simulink model "multi_model_attitude_controller1_1"  (R2016b)
settings: Solver=ode15s  StartTime=0.0  StopTime=inf  FixedStep=0.001  MaxStep=0.004  RelTol=1e-3
InitFcn:
  | kR_old=0;
  | kOm_old=0;
undefined symbols (not defined in the file or in its folder): deg, rad, s
libraries: simulink x32, aerolibconvert2 x6, aerolibobsolete x2, aerolibtransform2 x2, aerolibatmos2 x2, aerolibnav x2, aerolibanimutils x2
(part 1 of 3)
settings Model: Creator=ADAM  LastModifiedBy=luminghua
settings SolverCC: ExtrapolationOrder=1
settings DataIOCC: MaxDataPoints=1  SaveFormat=Structure  SignalLoggingSaveFormat=ModelDataLogs  SaveOutput=off  SignalLogging=off  DSMLogging=off  SaveTime=off  OutputSaveName=model_out  SignalLoggingName=model_out
settings OptimizationCC: ExpressionDepthLimit=2147483647  LifeSpan=inf  SimCompilerOptimization=on
settings DebuggingCC: UnderspecifiedInitializationDetection=Classic  MergeDetectMultiDrivingBlocksExec=none  SolverPrmCheckMsg=warning  InheritedTsInSrcMsg=none  MultiTaskDSMMsg=warning  MultiTaskCondExecSysMsg=none  FcnCallInpInsideContextMsg=warning  UnconnectedInputMsg=none  UnconnectedOutputMsg=none  UnconnectedLineMsg=none  AllowSymbolicDim=off  StateNameClashWarn=warning  SFUnexpectedBacktrackingDiag=warning  SFNoUnconditionalDefaultTransitionDiag=warning  SFExecutionAtInitializationDiag=none
settings HardwareCC: ProdBitPerPointer=32  ProdBitPerSizeT=32  ProdBitPerPtrDiffT=32  ProdLargestAtomicFloat=None  ProdWordSize=32  ProdHWDeviceType=Generic->32-bit x86 compatible
settings ModelReferenceCC: PropagateSignalLabelsOutOfModel=off
settings CodeAppCC: MaxIdLength=95
settings GRTTargetCC: TargetLangStandard=C89/C90 (ANSI)  GeneratePreprocessorConditionals=Disable all
settings ConfigComp: CovMetricSettings=dw  CovHtmlReporting=on  CovSaveCumulativeToWorkspaceVar=on  CovSaveSingleToWorkspaceVar=on  CovExternalEMLEnable=off

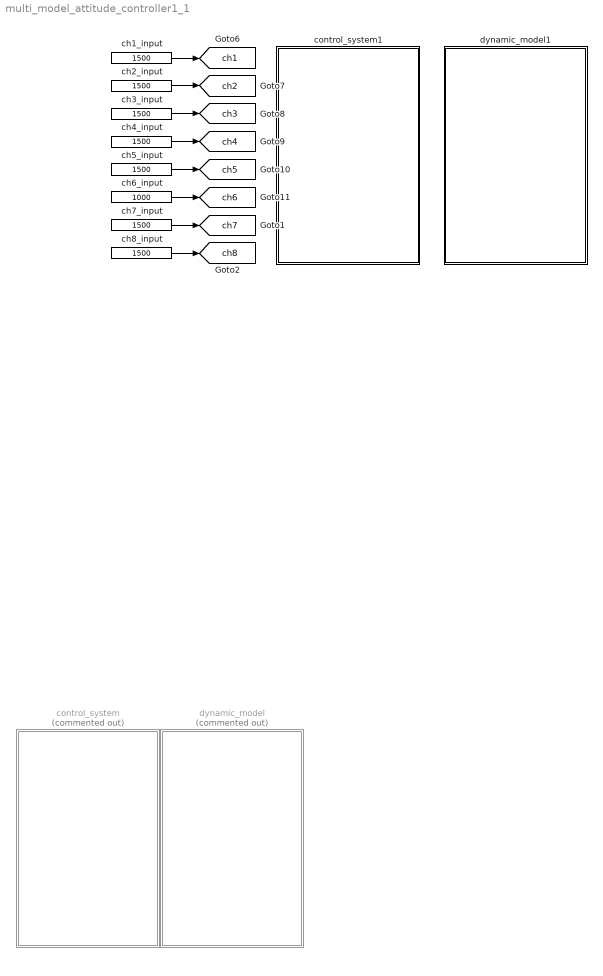
== system multi_model_attitude_controller1_1 ==
  ch1_input : Constant  Value=1500  SampleTime=0.004
  ch2_input : Constant  Value=1500  SampleTime=0.004
  ch3_input : Constant  Value=1500  SampleTime=0.004
  ch4_input : Constant  Value=1500  SampleTime=0.004
  ch5_input : Constant  Value=1500  SampleTime=0.004
  ch6_input : Constant  Value=1000  SampleTime=0.004
  ch7_input : Constant  Value=1500  SampleTime=0.004
  ch8_input : Constant  Value=1500  SampleTime=0.004
  control_system : Subsystem  Commented=on
      mask Display: fprintf('Embedded Software')
  control_system1 : Subsystem
      mask Display: fprintf('Embedded Software')
  dynamic_model : Subsystem  Commented=on
      mask Display: fprintf('Dynamic Model');
  dynamic_model1 : Subsystem
      mask Display: fprintf('Dynamic Model');
  tag scope: ch1=global, ch2=global, ch3=global, ch4=global, ch5=global, ch6=global, ch7=global, ch8=global
  wires:
  ch3_input/1 -> [ch3]
  ch2_input/1 -> [ch2]
  ch1_input/1 -> [ch1]
  ch4_input/1 -> [ch4]
  ch5_input/1 -> [ch5]
  ch6_input/1 -> [ch6]
  ch7_input/1 -> [ch7]
  ch8_input/1 -> [ch8]

== system multi_model_attitude_controller1_1/control_system ==
  Constant4 : Constant  Commented=on  Value=0.07  SampleTime=0.004
  Constant6 : Constant  Commented=on  Value=0  SampleTime=0.004
  Constant7 : Constant  Commented=on  Value=0  SampleTime=0.004
  Fcn2 : Fcn  Expr=(u - 1500) / 500
  Fcn5 : Fcn  Expr=(u - 1500) / 500
  Fcn6 : Fcn  Expr=(u - 1000) / 1000
  Fcn7 : Fcn  Expr=(u - 1500) / 500
  Mux : Mux  Inputs=3
  Saturation10 : Saturate  UpperLimit=1  LowerLimit=0
  Saturation7 : Saturate  UpperLimit=1  LowerLimit=-1
  Saturation8 : Saturate  UpperLimit=1  LowerLimit=-1
  Saturation9 : Saturate  UpperLimit=1  LowerLimit=-1
  Subsystem : Subsystem
      mask Display: disp('Test')
  Subsystem1 : Subsystem  Commented=on
      mask Display: disp('Attitude_controller distur');
  Subsystem2 : Subsystem  Commented=on
      mask Display: disp( 'Attitude_controller  PID')
  Subsystem3 : Subsystem
      mask Display: disp('Attitude_controller distur');
  tag scope: Moment=global
  wires:
  [ch1] -> Fcn2/1
  [ch2] -> Fcn5/1
  [ch4] -> Fcn7/1
  Fcn7/1 -> Saturation7/1
  Fcn5/1 -> Saturation8/1
  Fcn2/1 -> Saturation9/1
  [ch3] -> Fcn6/1
  Fcn6/1 -> Saturation10/1
  Subsystem1/1(M_roll) -> ?  "M_roll"
  Subsystem1/2(M_pitch) -> ?  "M_pitch"
  Subsystem1/3(M_yaw) -> ?  "M_yaw"
  Subsystem2/1(Out1) -> ?  "M_roll"
  Subsystem2/2(Out2) -> ?  "M_pitch"
  Subsystem2/3(Out3) -> ?  "M-yaw"
  Constant7/1 -> ?
  Constant6/1 -> ?
  Constant4/1 -> ?
  Subsystem3/1(M_roll) -> Mux/1
  Subsystem3/2(M_pitch) -> Mux/2
  Subsystem3/3(M_yaw) -> Mux/3
  Mux/1 -> [Moment]

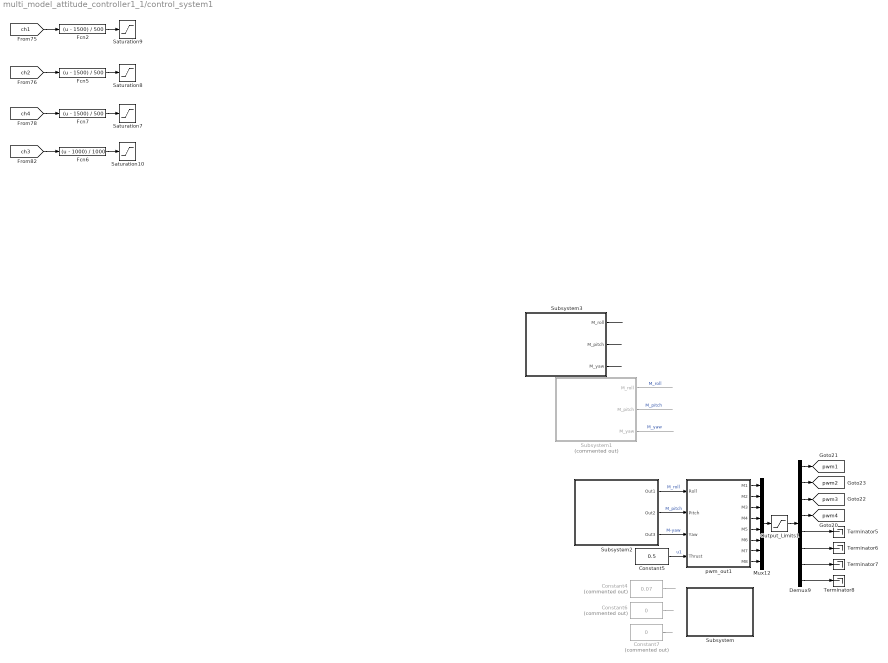
== system multi_model_attitude_controller1_1/control_system1 ==
  Constant4 : Constant  Commented=on  Value=0.07  SampleTime=0.004
  Constant5 : Constant  Value=0.5  SampleTime=0.004
  Constant6 : Constant  Commented=on  Value=0  SampleTime=0.004
  Constant7 : Constant  Commented=on  Value=0  SampleTime=0.004
  Demux9 : Demux  Outputs=8
  Fcn2 : Fcn  Expr=(u - 1500) / 500
  Fcn5 : Fcn  Expr=(u - 1500) / 500
  Fcn6 : Fcn  Expr=(u - 1000) / 1000
  Fcn7 : Fcn  Expr=(u - 1500) / 500
  Mux12 : Mux  Inputs=8
  Output_Limits1 : Saturate  UpperLimit=2000  LowerLimit=1000
  Saturation10 : Saturate  UpperLimit=1  LowerLimit=0
  Saturation7 : Saturate  UpperLimit=1  LowerLimit=-1
  Saturation8 : Saturate  UpperLimit=1  LowerLimit=-1
  Saturation9 : Saturate  UpperLimit=1  LowerLimit=-1
  Subsystem : Subsystem
      mask Display: disp('Test')
  Subsystem1 : Subsystem  Commented=on
      mask Display: disp('Attitude_controller distur');
  Subsystem2 : Subsystem
      mask Display: disp( 'Attitude_controller  PID')
  Subsystem3 : Subsystem
      mask Display: disp('Attitude_controller distur');
  Terminator{5..8} (4 alike) : Terminator
  pwm_out1 : MATLAB Function  TreatAsAtomicUnit=on  SystemSampleTime=0.004
  tag scope: pwm1=global, pwm2=global, pwm3=global, pwm4=global
  wires:
  pwm_out1/8(M8) -> Mux12/8
  pwm_out1/7(M7) -> Mux12/7
  pwm_out1/6(M6) -> Mux12/6
  pwm_out1/5(M5) -> Mux12/5
  pwm_out1/4(M4) -> Mux12/4
  pwm_out1/3(M3) -> Mux12/3
  pwm_out1/2(M2) -> Mux12/2
  pwm_out1/1(M1) -> Mux12/1
  Mux12/1 -> Output_Limits1/1
  [ch1] -> Fcn2/1
  [ch2] -> Fcn5/1
  [ch4] -> Fcn7/1
  Fcn7/1 -> Saturation7/1
  Fcn5/1 -> Saturation8/1
  Fcn2/1 -> Saturation9/1
  Demux9/5 -> Terminator5/1
  Demux9/6 -> Terminator6/1
  Demux9/7 -> Terminator7/1
  Demux9/8 -> Terminator8/1
  Demux9/1 -> [pwm1]
  Demux9/2 -> [pwm2]
  Demux9/3 -> [pwm3]
  Demux9/4 -> [pwm4]
  [ch3] -> Fcn6/1
  Fcn6/1 -> Saturation10/1
  Output_Limits1/1 -> Demux9/1
  Constant5/1 -> pwm_out1/4(Thrust)  "u1"
  Subsystem1/1(M_roll) -> ?  "M_roll"
  Subsystem1/2(M_pitch) -> ?  "M_pitch"
  Subsystem1/3(M_yaw) -> ?  "M_yaw"
  Subsystem2/1(Out1) -> pwm_out1/1(Roll)  "M_roll"
  Subsystem2/2(Out2) -> pwm_out1/2(Pitch)  "M_pitch"
  Subsystem2/3(Out3) -> pwm_out1/3(Yaw)  "M-yaw"
  Constant7/1 -> ?
  Constant6/1 -> ?
  Constant4/1 -> ?
  Subsystem3/1(M_roll) -> ?
  Subsystem3/2(M_pitch) -> ?
  Subsystem3/3(M_yaw) -> ?

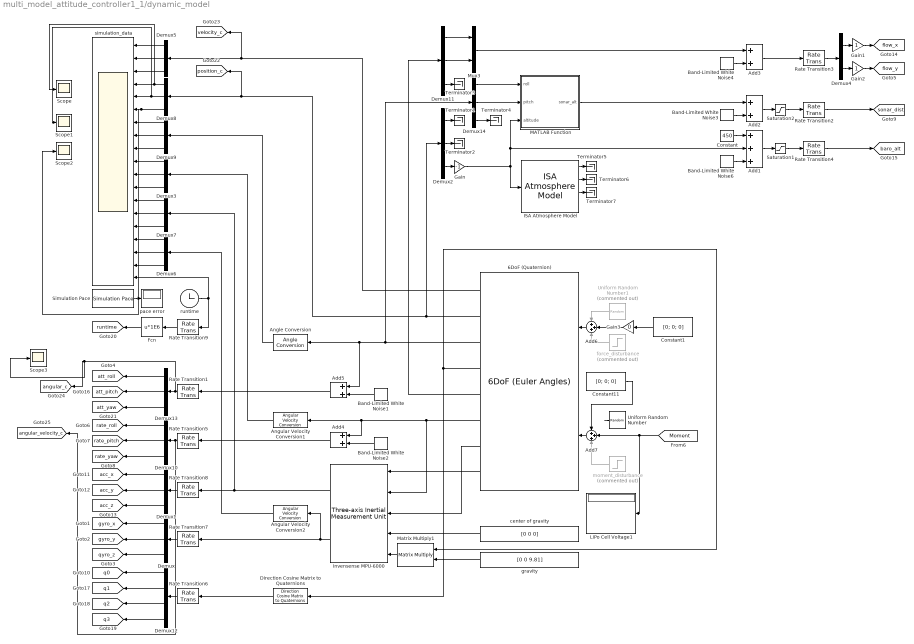
== system multi_model_attitude_controller1_1/dynamic_model ==
  6DoF (Quaternion) : aerolibobsolete/6DoF (Euler Angles)  units=Metric (MKS)  mtype=Fixed  rep=Quaternion  xme_0=[0 0 -1]  Vm_0=[0 0 0]  eul_0=[0 0 0]  pm_0=[0 0 0]  mass_0=0.26  mass_e=0  mass_f=0  inertia=[0.00080, 0, 0; 0, 0.00065, 0; 0, 0, 0.0014]  inertia_e=eye(3)  inertia_f=eye(3)  k_quat=1.0
  Add1 : Sum  Inputs=+++
  Add{2..5} (4 alike) : Sum
  Add6 : Sum  Inputs=+++
  Add7 : Sum  Inputs=+++
  Angle Conversion : aerolibconvert2/Angle Conversion  IU=rad  OU=deg
  Angular Velocity Conversion1 : aerolibconvert2/Angular Velocity Conversion  IU=rad/s  OU=deg/s
  Angular Velocity Conversion2 : aerolibconvert2/Angular Velocity Conversion  IU=rad/s  OU=deg/s
  Band-Limited White Noise1 : simulink/Sources/Band-Limited White Noise  Cov=0.00000000015  Ts=0.004  seed=[243584]
  Band-Limited White Noise2 : simulink/Sources/Band-Limited White Noise  Cov=0.000000002  Ts=0.004  seed=[243584]
  Band-Limited White Noise3 : simulink/Sources/Band-Limited White Noise  Cov=0.000005  Ts=0.1  seed=[31841]
  Band-Limited White Noise4 : simulink/Sources/Band-Limited White Noise  Cov=0.000000003  Ts=0.0067  seed=[25481]
  Band-Limited White Noise6 : simulink/Sources/Band-Limited White Noise  Cov=0.0005  Ts=0.008  seed=[79648]
  Constant : Constant  Value=450
  Constant1 : Constant  Value=[0; 0; 0]  SampleTime=5
  Constant11 : Constant  Value=[0; 0; 0]  SampleTime=5
  Demux{,1..3,5..11,13..14} (13 alike) : Demux  Outputs=3
  Demux12 : Demux
  Demux4 : Demux  Outputs=2
  Direction Cosine Matrix to Quaternions : aerolibtransform2/Direction Cosine Matrix  to Quaternions
  Fcn : Fcn  Expr=u*1E6
      mask Display: fprintf('uS');
  Gain : Gain  Gain=-1
  Gain1 : Gain
  Gain2 : Gain
  Gain3 : Gain  Gain=0
  ISA Atmosphere Model : aerolibatmos2/ISA Atmosphere Model  custom=on  g=9.80665  gamma=1.4  R=287.0531  L=0.0065  h_trop=11000  h_strat=20000  rho0=1.225  P0=101325  T0=288.15  h0=0
  Invensense MPU-6000 : aerolibnav/Three-axis Inertial Measurement Unit  units=Metric (MKS)  imu=[0 0 0]  i_Ts=0.004  dtype_a=off  w_a=190  z_a=0.707  a_sf_cc=[0.98 0 0; 0 0.98 0; 0 0 0.98]  a_bias=[0 0 0]  a_sat="[-19.62  -19.62  -19.62 19.62 19.62 19.62]"  dtype_g=off  w_g=190  z_g=0.707  g_sf_cc=[.98 0 0; 0 .98 0; 0 0 .98]  g_bias=[0 0 0]  g_sens=[0 0 0]  g_sat="[-4.36  -4.36  -4.36 4.36 4.36 4.36]"  i_rand=on  i_seeds=[348631 366719 978432 189621 128794 214632]  i_pow=[0.0000005 0.0000005 0.0000005 0.000000002 0.000000002 0.000000002]
  LiPo Cell Voltage1 : Display
  MATLAB Function : MATLAB Function  TreatAsAtomicUnit=on
  Matrix Multiply1 : Product  Multiplication=Matrix(*)
  Mux3 : Mux  Inputs=2
  Rate Transition{1,5..9} (6 alike) : RateTransition  OutPortSampleTime=0.004
  Rate Transition2 : RateTransition  OutPortSampleTime=0.1
  Rate Transition3 : RateTransition  OutPortSampleTime=0.0067
  Rate Transition4 : RateTransition  OutPortSampleTime=0.008
  Saturation1 : Saturate  UpperLimit=inf  LowerLimit=0
  Saturation2 : Saturate  UpperLimit=5  LowerLimit=0.3
  Scope{,1..3} (4 alike) : Scope
  Simulation Pace : aerolibanimutils/Simulation Pace  SimulationPace=1  SleepMode=MATLAB Thread  OutputPaceError=on  SampleTime=0.004
      settings: AttributesFormatString=%<SimulationPace> sec/sec
  Terminator{1..7} (7 alike) : Terminator
  Uniform Random Number : UniformRandomNumber  Minimum=[-0.0005 -0.0005 -0.0001]  Maximum=[0.5 0.0005 0.0001]  SampleTime=5
  Uniform Random Number1 : UniformRandomNumber  Commented=on  Minimum=[-0.01 -0.01 -0.1]  Maximum=[0.01 0.01 0.1]  SampleTime=5
  center of gravity : Constant  Value=[0 0 0]
  force_disturbance : Step  Commented=on  Time=5  Before=[0 0 0]  After=[0 0 0]
  gravity : Constant  Value=[0 0 9.81]
  moment_disturbance : Step  Commented=on  Time=5  Before=[0 0 0]  After=[0 0 0]
  pace error : Display
  runtime : Clock
  simulation_data : Scope  NumInputPorts=19
  tag scope: acc_x=global, acc_y=global, acc_z=global, angular_c=global, angular_velocity_c=global, att_pitch=global, att_roll=global, att_yaw=global, baro_alt=global, flow_x=global, flow_y=global, gyro_x=global, gyro_y=global, position_c=global, q0=global, q1=global, q2=global, q3=global, qyro_z=global, rate_pitch=global, rate_roll=global, rate_yaw=global, runtime=global, sonar_dist=global, velocity_c=global
  wires:
  6DoF (Quaternion)/7 -> Invensense MPU-6000/3
  Demux1/1 -> [acc_x]
  6DoF (Quaternion)/3 -> Demux14/1, Angle Conversion/1, Add5/1
  6DoF (Quaternion)/8 -> Invensense MPU-6000/1
  6DoF (Quaternion)/5 -> Demux11/1
  Demux9/1 -> simulation_data/7
  Demux9/2 -> simulation_data/8
  Demux3/1 -> simulation_data/10
  Demux3/2 -> simulation_data/11
  Demux3/3 -> simulation_data/12
  Demux7/1 -> simulation_data/13
  Demux7/2 -> simulation_data/14
  Demux7/3 -> simulation_data/15
  Demux/1 -> [gyro_x]
  Demux/2 -> [gyro_y]
  Demux/3 -> [qyro_z]
  Demux1/2 -> [acc_y]
  Demux5/1 -> simulation_data/1
  Demux5/2 -> simulation_data/2
  Demux5/3 -> simulation_data/3
  Demux8/1 -> Scope/1, simulation_data/4
  Demux8/2 -> Scope1/1, simulation_data/5
  Demux8/3 -> Scope2/1, simulation_data/6
  6DoF (Quaternion)/6 -> Invensense MPU-6000/2, Add4/1, Angular Velocity Conversion1/1
  Demux9/3 -> simulation_data/9
  Demux6/1 -> simulation_data/16
  Demux6/2 -> simulation_data/17
  Demux6/3 -> simulation_data/18
  Angular Velocity Conversion2/1 -> Demux6/1
  Demux1/3 -> [acc_z]
  Demux10/1 -> [rate_roll]
  Demux10/2 -> [rate_pitch]
  Demux10/3 -> [rate_yaw]
  Band-Limited White Noise2/1 -> Add4/2
  Add4/1 -> Rate Transition5/1
  Rate Transition5/1 -> [angular_velocity_c], Demux10/1
  6DoF (Quaternion)/4 -> Matrix Multiply1/1, Direction Cosine Matrix to Quaternions/1
  Simulation Pace/1 -> pace error/1
  6DoF (Quaternion)/1 -> Demux5/1, [velocity_c]
  6DoF (Quaternion)/2 -> Demux2/1, Demux8/1, [position_c]
  Angle Conversion/1 -> Demux9/1
  Angular Velocity Conversion1/1 -> Demux3/1
  Invensense MPU-6000/1 -> Rate Transition8/1, Demux7/1
  Invensense MPU-6000/2 -> Rate Transition7/1, Angular Velocity Conversion2/1
  runtime/1 -> simulation_data/19, Rate Transition9/1
  Rate Transition7/1 -> Demux/1
  Rate Transition8/1 -> Demux1/1
  Direction Cosine Matrix to Quaternions/1 -> Rate Transition6/1
  Rate Transition6/1 -> Demux12/1
  Demux12/4 -> [q3]
  Demux12/3 -> [q2]
  Demux12/2 -> [q1]
  Demux12/1 -> [q0]
  Fcn/1 -> [runtime]
  Rate Transition9/1 -> Fcn/1
  Demux13/1 -> [att_roll]
  Demux13/2 -> [att_pitch]
  Demux13/3 -> [att_yaw]
  Rate Transition1/1 -> Scope3/1, [angular_c], Demux13/1
  Band-Limited White Noise1/1 -> Add5/2
  Add5/1 -> Rate Transition1/1
  Add6/1 -> 6DoF (Quaternion)/1
  Add7/1 -> 6DoF (Quaternion)/2
  center of gravity/1 -> Invensense MPU-6000/4
  gravity/1 -> Matrix Multiply1/2
  Matrix Multiply1/1 -> Invensense MPU-6000/5
  moment_disturbance/1 -> Add7/3
  force_disturbance/1 -> Add6/3
  Constant1/1 -> Gain3/1
  Uniform Random Number1/1 -> Add6/1
  Uniform Random Number/1 -> ?
  Rate Transition3/1 -> Demux4/1
  Add3/1 -> Rate Transition3/1
  Demux2/3 -> Gain/1
  Gain/1 -> ISA Atmosphere Model/1, MATLAB Function/3(altitude), Add1/2
  Demux2/2 -> Terminator2/1
  Demux2/1 -> Terminator1/1
  Demux11/1 -> Mux3/1
  Demux11/2 -> Mux3/2
  Demux11/3 -> Terminator3/1
  Rate Transition2/1 -> [sonar_dist]
  Rate Transition4/1 -> [baro_alt]
  Saturation1/1 -> Rate Transition4/1
  Saturation2/1 -> Rate Transition2/1
  Add1/1 -> Saturation1/1
  MATLAB Function/1(sonar_alt) -> Add2/1
  Band-Limited White Noise3/1 -> Add2/2
  Add2/1 -> Saturation2/1
  Band-Limited White Noise4/1 -> Add3/2
  Band-Limited White Noise6/1 -> Add1/3
  Constant/1 -> Add1/1
  Mux3/1 -> Add3/1
  Demux4/2 -> Gain2/1
  Demux4/1 -> Gain1/1
  Gain1/1 -> [flow_x]
  Gain2/1 -> [flow_y]
  Demux14/2 -> MATLAB Function/2(pitch)
  Demux14/1 -> MATLAB Function/1(roll)
  Demux14/3 -> Terminator4/1
  ISA Atmosphere Model/3 -> Terminator7/1
  ISA Atmosphere Model/2 -> Terminator6/1
  ISA Atmosphere Model/1 -> Terminator5/1
  Constant11/1 -> Add7/1
  [Moment] -> Add7/2, LiPo Cell Voltage1/1
  Gain3/1 -> Add6/2

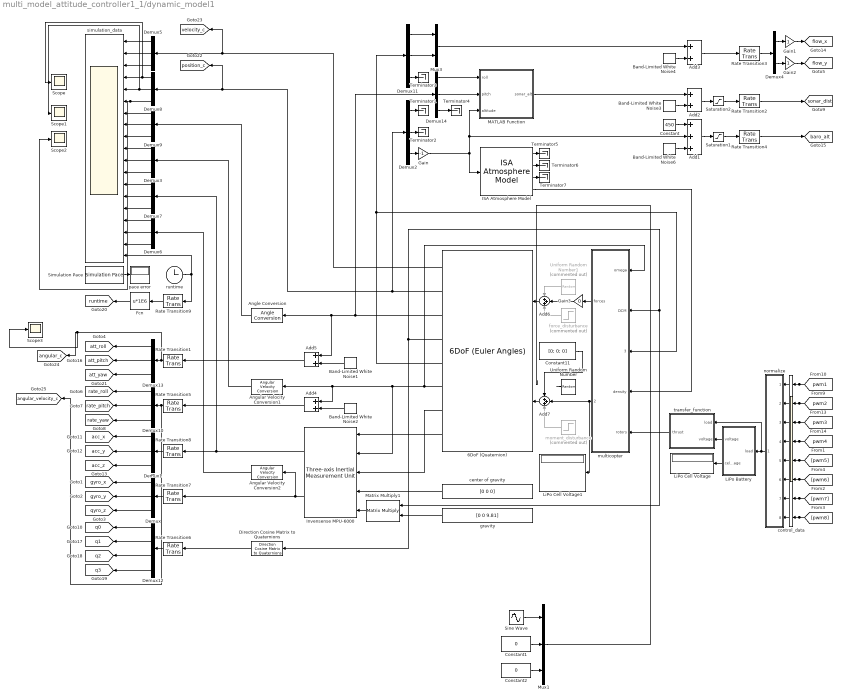
== system multi_model_attitude_controller1_1/dynamic_model1 ==
  6DoF (Quaternion) : aerolibobsolete/6DoF (Euler Angles)  units=Metric (MKS)  mtype=Fixed  rep=Quaternion  xme_0=[0 0 -1]  Vm_0=[0 0 0]  eul_0=[0 0 0]  pm_0=[0 0 0]  mass_0=0.26  mass_e=0  mass_f=0  inertia=[0.00080, 0, 0; 0, 0.00065, 0; 0, 0, 0.0014]  inertia_e=eye(3)  inertia_f=eye(3)  k_quat=1.0
  Add1 : Sum  Inputs=+++
  Add{2..5} (4 alike) : Sum
  Add6 : Sum  Inputs=+++
  Add7 : Sum  Inputs=+++
  Angle Conversion : aerolibconvert2/Angle Conversion  IU=rad  OU=deg
  Angular Velocity Conversion1 : aerolibconvert2/Angular Velocity Conversion  IU=rad/s  OU=deg/s
  Angular Velocity Conversion2 : aerolibconvert2/Angular Velocity Conversion  IU=rad/s  OU=deg/s
  Band-Limited White Noise1 : simulink/Sources/Band-Limited White Noise  Cov=0.00000000015  Ts=0.004  seed=[243584]
  Band-Limited White Noise2 : simulink/Sources/Band-Limited White Noise  Cov=0.000000002  Ts=0.004  seed=[243584]
  Band-Limited White Noise3 : simulink/Sources/Band-Limited White Noise  Cov=0.000005  Ts=0.1  seed=[31841]
  Band-Limited White Noise4 : simulink/Sources/Band-Limited White Noise  Cov=0.000000003  Ts=0.0067  seed=[25481]
  Band-Limited White Noise6 : simulink/Sources/Band-Limited White Noise  Cov=0.0005  Ts=0.008  seed=[79648]
  Constant : Constant  Value=450
  Constant1 : Constant  Value=0  SampleTime=0.004
  Constant11 : Constant  Value=[0; 0; 0]  SampleTime=5
  Constant2 : Constant  Value=0  SampleTime=0.004
  Demux{,1..3,5..11,13..14} (13 alike) : Demux  Outputs=3
  Demux12 : Demux
  Demux4 : Demux  Outputs=2
  Direction Cosine Matrix to Quaternions : aerolibtransform2/Direction Cosine Matrix  to Quaternions
  Fcn : Fcn  Expr=u*1E6
      mask Display: fprintf('uS');
  Gain : Gain  Gain=-1
  Gain1 : Gain
  Gain2 : Gain
  Gain3 : Gain  Gain=0
  ISA Atmosphere Model : aerolibatmos2/ISA Atmosphere Model  custom=on  g=9.80665  gamma=1.4  R=287.0531  L=0.0065  h_trop=11000  h_strat=20000  rho0=1.225  P0=101325  T0=288.15  h0=0
  Invensense MPU-6000 : aerolibnav/Three-axis Inertial Measurement Unit  units=Metric (MKS)  imu=[0 0 0]  i_Ts=0.004  dtype_a=off  w_a=190  z_a=0.707  a_sf_cc=[0.98 0 0; 0 0.98 0; 0 0 0.98]  a_bias=[0 0 0]  a_sat="[-19.62  -19.62  -19.62 19.62 19.62 19.62]"  dtype_g=off  w_g=190  z_g=0.707  g_sf_cc=[.98 0 0; 0 .98 0; 0 0 .98]  g_bias=[0 0 0]  g_sens=[0 0 0]  g_sat="[-4.36  -4.36  -4.36 4.36 4.36 4.36]"  i_rand=on  i_seeds=[348631 366719 978432 189621 128794 214632]  i_pow=[0.0000005 0.0000005 0.0000005 0.000000002 0.000000002 0.000000002]
  LiPo Battery : MATLAB Function  TreatAsAtomicUnit=on  SystemSampleTime=0.004
  LiPo Cell Voltage : Display
  LiPo Cell Voltage1 : Display
  MATLAB Function : MATLAB Function  TreatAsAtomicUnit=on
  Matrix Multiply1 : Product  Multiplication=Matrix(*)
  Mux1 : Mux  Inputs=3
  Mux3 : Mux  Inputs=2
  Rate Transition{1,5..9} (6 alike) : RateTransition  OutPortSampleTime=0.004
  Rate Transition2 : RateTransition  OutPortSampleTime=0.1
  Rate Transition3 : RateTransition  OutPortSampleTime=0.0067
  Rate Transition4 : RateTransition  OutPortSampleTime=0.008
  Saturation1 : Saturate  UpperLimit=inf  LowerLimit=0
  Saturation2 : Saturate  UpperLimit=5  LowerLimit=0.3
  Scope{,1..3} (4 alike) : Scope
  Simulation Pace : aerolibanimutils/Simulation Pace  SimulationPace=1  SleepMode=MATLAB Thread  OutputPaceError=on  SampleTime=0.004
      settings: AttributesFormatString=%<SimulationPace> sec/sec
  Sine Wave : Sin  Amplitude=0.5  Frequency=0.01  SampleTime=0.004
  Terminator{1..7} (7 alike) : Terminator
  Uniform Random Number : UniformRandomNumber  Minimum=[-0.0005 -0.0005 -0.0001]  Maximum=[0.5 0.0005 0.0001]  SampleTime=5
  Uniform Random Number1 : UniformRandomNumber  Commented=on  Minimum=[-0.01 -0.01 -0.1]  Maximum=[0.01 0.01 0.1]  SampleTime=5
  center of gravity : Constant  Value=[0 0 0]
  control_data : Scope  NumInputPorts=8
  force_disturbance : Step  Commented=on  Time=5  Before=[0 0 0]  After=[0 0 0]
  gravity : Constant  Value=[0 0 9.81]
  moment_disturbance : Step  Commented=on  Time=5  Before=[0 0 0]  After=[0 0 0]
  multicopter : MATLAB Function  TreatAsAtomicUnit=on
  normalize : Subsystem
      mask Display:
      | port_label('input', 1, 'pwm1');
      | port_label('input', 2, 'pwm2');
      | port_label('input', 3, 'pwm3');
      | port_label('input', 4, 'pwm4');
      | port_label('input', 5, 'pwm5');
      | port_label('input', 6, 'pwm6');
      | port_label('input', 7, 'pwm7');
      | port_label('input', 8, 'pwm8');
  pace error : Display
  runtime : Clock
  simulation_data : Scope  NumInputPorts=19
  transfer_function : Subsystem
      mask Display: fprintf('Brushless Motors')
  tag scope: acc_x=global, acc_y=global, acc_z=global, angular_c=global, angular_velocity_c=global, att_pitch=global, att_roll=global, att_yaw=global, baro_alt=global, flow_x=global, flow_y=global, gyro_x=global, gyro_y=global, position_c=global, q0=global, q1=global, q2=global, q3=global, qyro_z=global, rate_pitch=global, rate_roll=global, rate_yaw=global, runtime=global, sonar_dist=global, velocity_c=global
  wires:
  6DoF (Quaternion)/7 -> Invensense MPU-6000/3
  Demux1/1 -> [acc_x]
  6DoF (Quaternion)/3 -> Demux14/1, Angle Conversion/1, Add5/1
  6DoF (Quaternion)/8 -> Invensense MPU-6000/1
  6DoF (Quaternion)/5 -> Demux11/1, multicopter/3(velocity)
  Demux9/1 -> simulation_data/7
  Demux9/2 -> simulation_data/8
  Demux3/1 -> simulation_data/10
  Demux3/2 -> simulation_data/11
  Demux3/3 -> simulation_data/12
  Demux7/1 -> simulation_data/13
  Demux7/2 -> simulation_data/14
  Demux7/3 -> simulation_data/15
  Demux/1 -> [gyro_x]
  Demux/2 -> [gyro_y]
  Demux/3 -> [qyro_z]
  Demux1/2 -> [acc_y]
  Demux5/1 -> simulation_data/1
  Demux5/2 -> simulation_data/2
  Demux5/3 -> simulation_data/3
  Demux8/1 -> Scope/1, simulation_data/4
  Demux8/2 -> Scope1/1, simulation_data/5
  Demux8/3 -> Scope2/1, simulation_data/6
  6DoF (Quaternion)/6 -> multicopter/1(omega), Invensense MPU-6000/2, Add4/1, Angular Velocity Conversion1/1
  Demux9/3 -> simulation_data/9
  Demux6/1 -> simulation_data/16
  Demux6/2 -> simulation_data/17
  Demux6/3 -> simulation_data/18
  Angular Velocity Conversion2/1 -> Demux6/1
  Demux1/3 -> [acc_z]
  Demux10/1 -> [rate_roll]
  Demux10/2 -> [rate_pitch]
  Demux10/3 -> [rate_yaw]
  Band-Limited White Noise2/1 -> Add4/2
  Add4/1 -> Rate Transition5/1
  Rate Transition5/1 -> [angular_velocity_c], Demux10/1
  6DoF (Quaternion)/4 -> Matrix Multiply1/1, multicopter/2(DCM), Direction Cosine Matrix to Quaternions/1
  Simulation Pace/1 -> pace error/1
  6DoF (Quaternion)/1 -> Demux5/1, [velocity_c]
  6DoF (Quaternion)/2 -> Demux2/1, Demux8/1, [position_c]
  Angle Conversion/1 -> Demux9/1
  Angular Velocity Conversion1/1 -> Demux3/1
  Invensense MPU-6000/1 -> Rate Transition8/1, Demux7/1
  Invensense MPU-6000/2 -> Rate Transition7/1, Angular Velocity Conversion2/1
  runtime/1 -> simulation_data/19, Rate Transition9/1
  Rate Transition7/1 -> Demux/1
  Rate Transition8/1 -> Demux1/1
  Direction Cosine Matrix to Quaternions/1 -> Rate Transition6/1
  Rate Transition6/1 -> Demux12/1
  [pwm1] -> normalize/1(pwm1), control_data/1
  [pwm2] -> normalize/2(pwm2), control_data/2
  [pwm3] -> normalize/3(pwm3), control_data/3
  [pwm4] -> normalize/4(pwm4), control_data/4
  [pwm5] -> normalize/5(pwm5), control_data/5
  [pwm6] -> normalize/6(pwm6), control_data/6
  [pwm7] -> normalize/7(pwm7), control_data/7
  [pwm8] -> normalize/8(pwm8), control_data/8
  Demux12/4 -> [q3]
  Demux12/3 -> [q2]
  Demux12/2 -> [q1]
  Demux12/1 -> [q0]
  Fcn/1 -> [runtime]
  Rate Transition9/1 -> Fcn/1
  normalize/1(normalized_signals) -> transfer_function/1(load), LiPo Battery/1(load)
  LiPo Battery/1(voltage) -> transfer_function/2(voltage)
  transfer_function/1(thrust) -> multicopter/5(rotors)
  LiPo Battery/2(cell_voltage) -> LiPo Cell Voltage/1
  Demux13/1 -> [att_roll]
  Demux13/2 -> [att_pitch]
  Demux13/3 -> [att_yaw]
  Rate Transition1/1 -> Scope3/1, [angular_c], Demux13/1
  Band-Limited White Noise1/1 -> Add5/2
  Add5/1 -> Rate Transition1/1
  Add6/1 -> 6DoF (Quaternion)/1
  Add7/1 -> 6DoF (Quaternion)/2
  center of gravity/1 -> Invensense MPU-6000/4
  gravity/1 -> Matrix Multiply1/2
  Matrix Multiply1/1 -> Invensense MPU-6000/5
  moment_disturbance/1 -> Add7/3
  force_disturbance/1 -> Add6/3
  multicopter/1(forces) -> Gain3/1
  Uniform Random Number1/1 -> Add6/1
  Uniform Random Number/1 -> ?
  Rate Transition3/1 -> Demux4/1
  Add3/1 -> Rate Transition3/1
  Demux2/3 -> Gain/1
  Gain/1 -> ISA Atmosphere Model/1, MATLAB Function/3(altitude), Add1/2
  Demux2/2 -> Terminator2/1
  Demux2/1 -> Terminator1/1
  Demux11/1 -> Mux3/1
  Demux11/2 -> Mux3/2
  Demux11/3 -> Terminator3/1
  Rate Transition2/1 -> [sonar_dist]
  Rate Transition4/1 -> [baro_alt]
  Saturation1/1 -> Rate Transition4/1
  Saturation2/1 -> Rate Transition2/1
  Add1/1 -> Saturation1/1
  MATLAB Function/1(sonar_alt) -> Add2/1
  Band-Limited White Noise3/1 -> Add2/2
  Add2/1 -> Saturation2/1
  Band-Limited White Noise4/1 -> Add3/2
  Band-Limited White Noise6/1 -> Add1/3
  Constant/1 -> Add1/1
  Mux3/1 -> Add3/1
  Demux4/2 -> Gain2/1
  Demux4/1 -> Gain1/1
  Gain1/1 -> [flow_x]
  Gain2/1 -> [flow_y]
  Demux14/2 -> MATLAB Function/2(pitch)
  Demux14/1 -> MATLAB Function/1(roll)
  Demux14/3 -> Terminator4/1
  ISA Atmosphere Model/3 -> Terminator7/1
  ISA Atmosphere Model/2 -> Terminator6/1
  ISA Atmosphere Model/1 -> Terminator5/1
  ISA Atmosphere Model/4 -> multicopter/4(density)
  Constant11/1 -> Add7/1
  multicopter/2(moments) -> Add7/2, LiPo Cell Voltage1/1
  Gain3/1 -> Add6/2
  Sine Wave/1 -> Mux1/1
  Constant1/1 -> Mux1/2
  Constant2/1 -> Mux1/3
  Mux1/1 -> ?

== system multi_model_attitude_controller1_1/control_system/Subsystem ==
  Add1 : Sum  Commented=on  Inputs=-+
  Add2 : Sum  Commented=on  Inputs=+-
  Constant : Constant  Commented=on  Value=[1 0 0]
  Constant1 : Constant  Commented=on  Value=[0 0 0]
  Constant11 : Constant  Value=[1; -1; 1]  SampleTime=0.004
  Constant9 : Constant  Value=[0.00080, 0, 0; 0, 0.00065, 0; 0, 0, 0.0014]  SampleTime=0.004
  Display10 : Display  Commented=on
  Display4 : Display
  Display5 : Display
  Display6 : Display
  Gain : Gain  Commented=on  Gain=1/2
  MATLAB Function3 : MATLAB Function  Commented=on  TreatAsAtomicUnit=on
  MATLAB Function4 : MATLAB Function  Commented=on  TreatAsAtomicUnit=on
  MATLAB Function5 : MATLAB Function  Commented=on  TreatAsAtomicUnit=on
  MATLAB Function7 : MATLAB Function  Commented=on  TreatAsAtomicUnit=on
  MATLAB Function8 : MATLAB Function  Commented=on  TreatAsAtomicUnit=on
  Product : Product  Inputs=/  Multiplication=Matrix(*)
  Product1 : Product  Multiplication=Matrix(*)
  Product3 : Product  Multiplication=Matrix(*)
  wires:
  ? -> Add2/1
  ? -> MATLAB Function3/1(angular)
  MATLAB Function7/1(RR) -> Add1/2
  Add1/1 -> MATLAB Function5/1(RdR_RRd)
  Constant/1 -> MATLAB Function4/1(angular)
  Gain/1 -> Display10/1  "err_R"
  MATLAB Function3/1(R) -> MATLAB Function8/1(a), MATLAB Function7/2(b)  "R"
  MATLAB Function5/1(err_R) -> Gain/1
  MATLAB Function8/1(RR) -> Add1/1
  MATLAB Function4/1(R) -> MATLAB Function8/2(b), MATLAB Function7/1(a)
  Constant1/1 -> Add2/2
  Product/1 -> Product1/1, Display5/1
  Constant11/1 -> Product3/2
  Constant9/1 -> Product3/1, Product1/2, Product/1
  Add2/1 -> ?  "err_W"
  Product3/1 -> Display6/1
  Product1/1 -> Display4/1

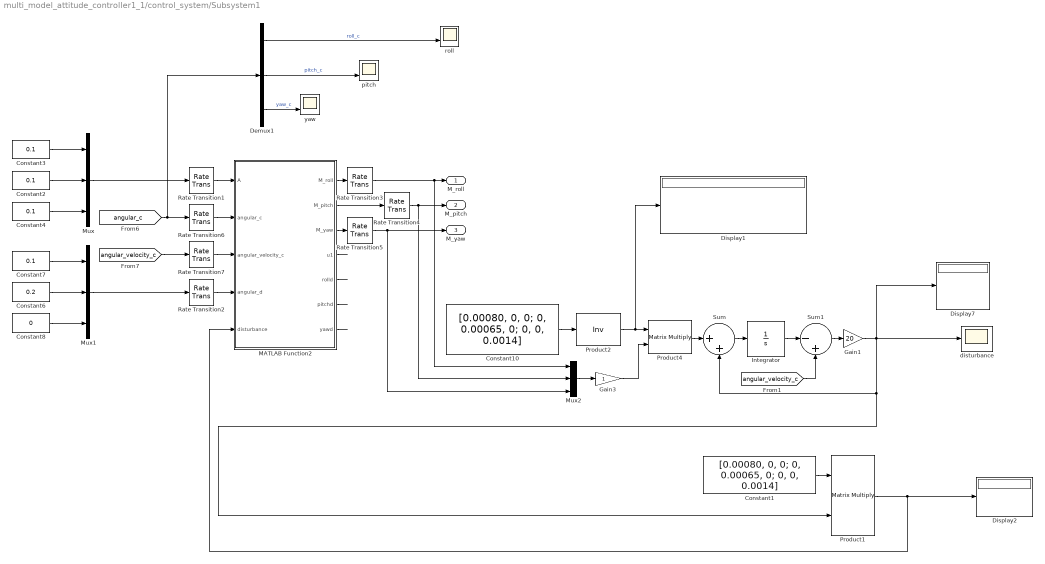
== system multi_model_attitude_controller1_1/control_system/Subsystem1 ==
  Constant1 : Constant  Value=[0.00080, 0, 0; 0, 0.00065, 0; 0, 0, 0.0014]  SampleTime=0.004
  Constant10 : Constant  Value=[0.00080, 0, 0; 0, 0.00065, 0; 0, 0, 0.0014]  SampleTime=0.004
  Constant{2..4,7} (4 alike) : Constant  Value=0.1  SampleTime=0.004
  Constant6 : Constant  Value=0.2  SampleTime=0.004
  Constant8 : Constant  Value=0  SampleTime=0.004
  Demux1 : Demux  Outputs=3
  Display1 : Display
  Display2 : Display
  Display7 : Display
  Gain1 : Gain  Gain=20
  Gain3 : Gain
  Integrator : Integrator
  MATLAB Function2 : MATLAB Function  TreatAsAtomicUnit=on
  Mux : Mux  Inputs=3
  Mux1 : Mux  Inputs=3
  Mux2 : Mux  Inputs=3
  Product1 : Product  Multiplication=Matrix(*)
  Product2 : Product  Inputs=/  Multiplication=Matrix(*)
  Product4 : Product  Multiplication=Matrix(*)
  Rate Transition{1..7} (7 alike) : RateTransition  OutPortSampleTime=0.004
  Sum : Sum  Inputs=|++
  Sum1 : Sum  Inputs=|-+
  disturbance : Scope
  pitch : Scope  NumInputPorts=2
  roll : Scope  NumInputPorts=2
  yaw : Scope  NumInputPorts=2
  M_roll : Outport
  M_pitch : Outport  Port=2
  M_yaw : Outport  Port=3
  wires:
  MATLAB Function2/4(u1) -> ?
  MATLAB Function2/6(pitchd) -> ?
  MATLAB Function2/7(yawd) -> ?
  MATLAB Function2/5(rolld) -> ?
  ? -> pitch/1
  ? -> roll/1
  ? -> yaw/1
  Demux1/2 -> pitch/2  "pitch_c"
  [angular_c] -> Demux1/1, Rate Transition6/1
  [angular_velocity_c] -> Rate Transition7/1
  Rate Transition1/1 -> MATLAB Function2/1(A)
  Demux1/1 -> roll/2  "roll_c"
  Rate Transition7/1 -> MATLAB Function2/3(angular_velocity_c)
  Demux1/3 -> yaw/2  "yaw_c"
  Rate Transition6/1 -> MATLAB Function2/2(angular_c)
  Integrator/1 -> Sum1/1
  Mux2/1 -> Gain3/1
  Constant4/1 -> Mux/3
  Mux1/1 -> Rate Transition2/1
  MATLAB Function2/2(M_pitch) -> Rate Transition4/1
  Constant3/1 -> Mux/1
  Product4/1 -> Sum/1
  Sum/1 -> Integrator/1
  MATLAB Function2/1(M_roll) -> Rate Transition3/1
  Sum1/1 -> Gain1/1
  Constant8/1 -> Mux1/3
  MATLAB Function2/3(M_yaw) -> Rate Transition5/1
  Product2/1 -> Display1/1, Product4/1
  Constant10/1 -> Product2/1
  Mux/1 -> Rate Transition1/1
  Gain1/1 -> Product1/2, Sum/2, disturbance/1, Display7/1
  [angular_velocity_c] -> Sum1/2
  Constant6/1 -> Mux1/2
  Constant7/1 -> Mux1/1
  Constant2/1 -> Mux/2
  Rate Transition2/1 -> MATLAB Function2/4(angular_d)
  Constant1/1 -> Product1/1
  Rate Transition3/1 -> Mux2/1, M_roll/1
  Rate Transition4/1 -> Mux2/2, M_pitch/1
  Rate Transition5/1 -> Mux2/3, M_yaw/1
  Product1/1 -> MATLAB Function2/5(disturbance), Display2/1
  Gain3/1 -> Product4/2

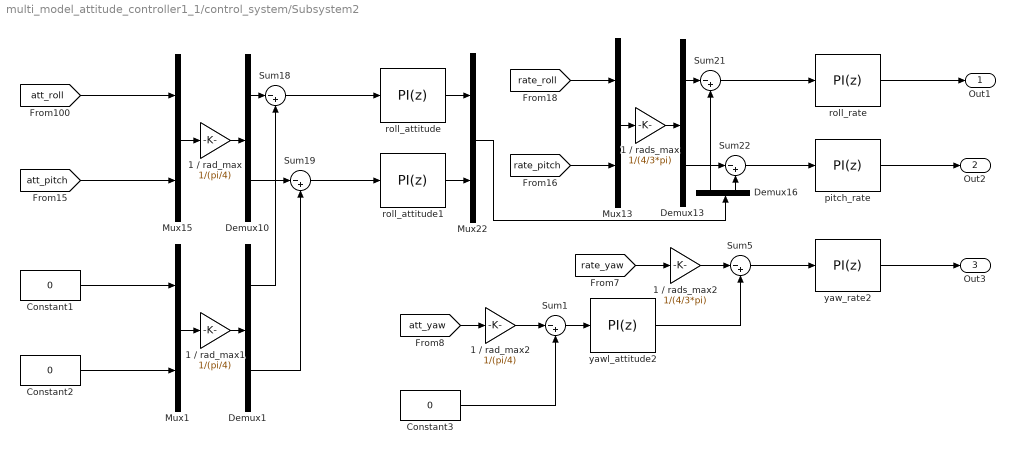
== system multi_model_attitude_controller1_1/control_system/Subsystem2 ==
  1 / rad_max : Gain  Gain=1/(pi/4)
  1 / rad_max1 : Gain  Gain=1/(pi/4)
  1 / rad_max2 : Gain  Gain=1/(pi/4)
  1 / rads_max : Gain  Gain=1/(4/3*pi)
  1 / rads_max2 : Gain  Gain=1/(4/3*pi)
  Constant1 : Constant  Value=0  SampleTime=0.004
  Constant2 : Constant  Value=0  SampleTime=0.004
  Constant3 : Constant  Value=0  SampleTime=0.004
  Demux{1,10,13,16} (4 alike) : Demux  Outputs=2
  Mux{1,13,15,22} (4 alike) : Mux  Inputs=2
  Sum{1,5,18..19,21..22} (6 alike) : Sum  Inputs=|-+
  pitch_rate : simulink/Continuous/PID Controller  Controller=PI  TimeDomain=Discrete-time  SampleTime=-1  IntegratorMethod=Forward Euler  FilterMethod=Forward Euler  Form=Parallel  UseFilter=on  ControllerParametersSource=internal  P=0.3  I=0.03  D=0.0024  N=100  InitialConditionSource=internal  InitialConditionForIntegrator=0  InitialConditionForFilter=0  ExternalReset=none  LimitOutput=on  UpperSaturationLimit=1  LowerSaturationLimit=-1  LinearizeAsGain=on  AntiWindupMode=none  Kb=1  TrackingMode=off  Kt=1  PParamMin=[]  PParamMax=[]  IParamMin=[]  IParamMax=[]  DParamMin=[]  DParamMax=[]  NParamMin=[]  NParamMax=[]  KbParamMin=[]  KbParamMax=[]  KtParamMin=[]  KtParamMax=[]  POutMin=[]  POutMax=[]  IOutMin=[]  IOutMax=[]  DOutMin=[]  DOutMax=[]  NOutMin=[]  NOutMax=[]  KbOutMin=[]  KbOutMax=[]  KtOutMin=[]  KtOutMax=[]  IntegratorOutMin=[]  IntegratorOutMax=[]  FilterOutMin=[]  FilterOutMax=[]  SumOutMin=[]  SumOutMax=[]  SumI1OutMin=[]  SumI1OutMax=[]  SumI2OutMin=[]  SumI2OutMax=[]  SumI3OutMin=[]  SumI3OutMax=[]  SumDOutMin=[]  SumDOutMax=[]  SaturationOutMin=[]  SaturationOutMax=[]  IntegratorContinuousStateAttributes=''  IntegratorStateMustResolveToSignalObject=off  IntegratorRTWStateStorageClass=Auto  FilterContinuousStateAttributes=''  FilterStateMustResolveToSignalObject=off  FilterRTWStateStorageClass=Auto  DifferentiatorICPrevScaledInput=0  DifferentiatorOutMin=[]  DifferentiatorOutMax=[]
  roll_attitude : simulink/Continuous/PID Controller  Controller=PI  TimeDomain=Discrete-time  SampleTime=-1  IntegratorMethod=Forward Euler  FilterMethod=Forward Euler  Form=Parallel  UseFilter=on  ControllerParametersSource=internal  P=1.23566755839648  I=1.81217768520031  D=0.01  N=100  InitialConditionSource=internal  InitialConditionForIntegrator=0  InitialConditionForFilter=0  ExternalReset=none  LimitOutput=on  UpperSaturationLimit=1  LowerSaturationLimit=-1  LinearizeAsGain=on  AntiWindupMode=none  Kb=1  TrackingMode=off  Kt=1  PParamMin=[]  PParamMax=[]  IParamMin=[]  IParamMax=[]  DParamMin=[]  DParamMax=[]  NParamMin=[]  NParamMax=[]  KbParamMin=[]  KbParamMax=[]  KtParamMin=[]  KtParamMax=[]  POutMin=[]  POutMax=[]  IOutMin=[]  IOutMax=[]  DOutMin=[]  DOutMax=[]  NOutMin=[]  NOutMax=[]  KbOutMin=[]  KbOutMax=[]  KtOutMin=[]  KtOutMax=[]  IntegratorOutMin=[]  IntegratorOutMax=[]  FilterOutMin=[]  FilterOutMax=[]  SumOutMin=[]  SumOutMax=[]  SumI1OutMin=[]  SumI1OutMax=[]  SumI2OutMin=[]  SumI2OutMax=[]  SumI3OutMin=[]  SumI3OutMax=[]  SumDOutMin=[]  SumDOutMax=[]  SaturationOutMin=[]  SaturationOutMax=[]  IntegratorContinuousStateAttributes=''  IntegratorStateMustResolveToSignalObject=off  IntegratorRTWStateStorageClass=Auto  FilterContinuousStateAttributes=''  FilterStateMustResolveToSignalObject=off  FilterRTWStateStorageClass=Auto  DifferentiatorICPrevScaledInput=0  DifferentiatorOutMin=[]  DifferentiatorOutMax=[]
  roll_attitude1 : simulink/Continuous/PID Controller  Controller=PI  TimeDomain=Discrete-time  SampleTime=-1  IntegratorMethod=Forward Euler  FilterMethod=Forward Euler  Form=Parallel  UseFilter=on  ControllerParametersSource=internal  P=0.5  I=0.05  D=0.01  N=100  InitialConditionSource=internal  InitialConditionForIntegrator=0  InitialConditionForFilter=0  ExternalReset=none  LimitOutput=on  UpperSaturationLimit=1  LowerSaturationLimit=-1  LinearizeAsGain=on  AntiWindupMode=none  Kb=1  TrackingMode=off  Kt=1  PParamMin=[]  PParamMax=[]  IParamMin=[]  IParamMax=[]  DParamMin=[]  DParamMax=[]  NParamMin=[]  NParamMax=[]  KbParamMin=[]  KbParamMax=[]  KtParamMin=[]  KtParamMax=[]  POutMin=[]  POutMax=[]  IOutMin=[]  IOutMax=[]  DOutMin=[]  DOutMax=[]  NOutMin=[]  NOutMax=[]  KbOutMin=[]  KbOutMax=[]  KtOutMin=[]  KtOutMax=[]  IntegratorOutMin=[]  IntegratorOutMax=[]  FilterOutMin=[]  FilterOutMax=[]  SumOutMin=[]  SumOutMax=[]  SumI1OutMin=[]  SumI1OutMax=[]  SumI2OutMin=[]  SumI2OutMax=[]  SumI3OutMin=[]  SumI3OutMax=[]  SumDOutMin=[]  SumDOutMax=[]  SaturationOutMin=[]  SaturationOutMax=[]  IntegratorContinuousStateAttributes=''  IntegratorStateMustResolveToSignalObject=off  IntegratorRTWStateStorageClass=Auto  FilterContinuousStateAttributes=''  FilterStateMustResolveToSignalObject=off  FilterRTWStateStorageClass=Auto  DifferentiatorICPrevScaledInput=0  DifferentiatorOutMin=[]  DifferentiatorOutMax=[]
  roll_rate : simulink/Continuous/PID Controller  Controller=PI  TimeDomain=Discrete-time  SampleTime=-1  IntegratorMethod=Forward Euler  FilterMethod=Forward Euler  Form=Parallel  UseFilter=on  ControllerParametersSource=internal  P=0.42490099698384  I=3.70850302525657  D=0.0024  N=100  InitialConditionSource=internal  InitialConditionForIntegrator=0  InitialConditionForFilter=0  ExternalReset=none  LimitOutput=on  UpperSaturationLimit=1  LowerSaturationLimit=-1  LinearizeAsGain=on  AntiWindupMode=none  Kb=1  TrackingMode=off  Kt=1  PParamMin=[]  PParamMax=[]  IParamMin=[]  IParamMax=[]  DParamMin=[]  DParamMax=[]  NParamMin=[]  NParamMax=[]  KbParamMin=[]  KbParamMax=[]  KtParamMin=[]  KtParamMax=[]  POutMin=[]  POutMax=[]  IOutMin=[]  IOutMax=[]  DOutMin=[]  DOutMax=[]  NOutMin=[]  NOutMax=[]  KbOutMin=[]  KbOutMax=[]  KtOutMin=[]  KtOutMax=[]  IntegratorOutMin=[]  IntegratorOutMax=[]  FilterOutMin=[]  FilterOutMax=[]  SumOutMin=[]  SumOutMax=[]  SumI1OutMin=[]  SumI1OutMax=[]  SumI2OutMin=[]  SumI2OutMax=[]  SumI3OutMin=[]  SumI3OutMax=[]  SumDOutMin=[]  SumDOutMax=[]  SaturationOutMin=[]  SaturationOutMax=[]  IntegratorContinuousStateAttributes=''  IntegratorStateMustResolveToSignalObject=off  IntegratorRTWStateStorageClass=Auto  FilterContinuousStateAttributes=''  FilterStateMustResolveToSignalObject=off  FilterRTWStateStorageClass=Auto  DifferentiatorICPrevScaledInput=0  DifferentiatorOutMin=[]  DifferentiatorOutMax=[]
  yaw_rate2 : simulink/Continuous/PID Controller  Controller=PI  TimeDomain=Discrete-time  SampleTime=-1  IntegratorMethod=Forward Euler  FilterMethod=Forward Euler  Form=Parallel  UseFilter=on  ControllerParametersSource=internal  P=0.3  I=0.03  D=0.0024  N=100  InitialConditionSource=internal  InitialConditionForIntegrator=0  InitialConditionForFilter=0  ExternalReset=none  LimitOutput=on  UpperSaturationLimit=1  LowerSaturationLimit=-1  LinearizeAsGain=on  AntiWindupMode=none  Kb=1  TrackingMode=off  Kt=1  PParamMin=[]  PParamMax=[]  IParamMin=[]  IParamMax=[]  DParamMin=[]  DParamMax=[]  NParamMin=[]  NParamMax=[]  KbParamMin=[]  KbParamMax=[]  KtParamMin=[]  KtParamMax=[]  POutMin=[]  POutMax=[]  IOutMin=[]  IOutMax=[]  DOutMin=[]  DOutMax=[]  NOutMin=[]  NOutMax=[]  KbOutMin=[]  KbOutMax=[]  KtOutMin=[]  KtOutMax=[]  IntegratorOutMin=[]  IntegratorOutMax=[]  FilterOutMin=[]  FilterOutMax=[]  SumOutMin=[]  SumOutMax=[]  SumI1OutMin=[]  SumI1OutMax=[]  SumI2OutMin=[]  SumI2OutMax=[]  SumI3OutMin=[]  SumI3OutMax=[]  SumDOutMin=[]  SumDOutMax=[]  SaturationOutMin=[]  SaturationOutMax=[]  IntegratorContinuousStateAttributes=''  IntegratorStateMustResolveToSignalObject=off  IntegratorRTWStateStorageClass=Auto  FilterContinuousStateAttributes=''  FilterStateMustResolveToSignalObject=off  FilterRTWStateStorageClass=Auto  DifferentiatorICPrevScaledInput=0  DifferentiatorOutMin=[]  DifferentiatorOutMax=[]
  yawl_attitude2 : simulink/Continuous/PID Controller  Controller=PI  TimeDomain=Discrete-time  SampleTime=-1  IntegratorMethod=Forward Euler  FilterMethod=Forward Euler  Form=Parallel  UseFilter=on  ControllerParametersSource=internal  P=0.5  I=0.05  D=0.01  N=100  InitialConditionSource=internal  InitialConditionForIntegrator=0  InitialConditionForFilter=0  ExternalReset=none  LimitOutput=on  UpperSaturationLimit=1  LowerSaturationLimit=-1  LinearizeAsGain=on  AntiWindupMode=none  Kb=1  TrackingMode=off  Kt=1  PParamMin=[]  PParamMax=[]  IParamMin=[]  IParamMax=[]  DParamMin=[]  DParamMax=[]  NParamMin=[]  NParamMax=[]  KbParamMin=[]  KbParamMax=[]  KtParamMin=[]  KtParamMax=[]  POutMin=[]  POutMax=[]  IOutMin=[]  IOutMax=[]  DOutMin=[]  DOutMax=[]  NOutMin=[]  NOutMax=[]  KbOutMin=[]  KbOutMax=[]  KtOutMin=[]  KtOutMax=[]  IntegratorOutMin=[]  IntegratorOutMax=[]  FilterOutMin=[]  FilterOutMax=[]  SumOutMin=[]  SumOutMax=[]  SumI1OutMin=[]  SumI1OutMax=[]  SumI2OutMin=[]  SumI2OutMax=[]  SumI3OutMin=[]  SumI3OutMax=[]  SumDOutMin=[]  SumDOutMax=[]  SaturationOutMin=[]  SaturationOutMax=[]  IntegratorContinuousStateAttributes=''  IntegratorStateMustResolveToSignalObject=off  IntegratorRTWStateStorageClass=Auto  FilterContinuousStateAttributes=''  FilterStateMustResolveToSignalObject=off  FilterRTWStateStorageClass=Auto  DifferentiatorICPrevScaledInput=0  DifferentiatorOutMin=[]  DifferentiatorOutMax=[]
  Out1 : Outport
  Out2 : Outport  Port=2
  Out3 : Outport  Port=3
  wires:
  Constant1/1 -> Mux1/1
  Mux1/1 -> 1 / rad_max1/1
  Constant2/1 -> Mux1/2
  Demux1/1 -> Sum18/2
  Mux22/1 -> Demux16/1
  yaw_rate2/1 -> Out3/1
  Sum5/1 -> yaw_rate2/1
  yawl_attitude2/1 -> Sum5/2
  1 / rad_max2/1 -> Sum1/1
  [att_yaw] -> 1 / rad_max2/1
  1 / rads_max2/1 -> Sum5/1
  [rate_yaw] -> 1 / rads_max2/1
  1 / rad_max/1 -> Demux10/1
  Demux10/1 -> Sum18/1
  Demux16/2 -> Sum22/2
  roll_attitude1/1 -> Mux22/2
  Demux13/2 -> Sum22/1
  Sum21/1 -> roll_rate/1
  Sum22/1 -> pitch_rate/1
  roll_attitude/1 -> Mux22/1
  [rate_pitch] -> Mux13/2
  Demux10/2 -> Sum19/1
  [att_pitch] -> Mux15/2
  [rate_roll] -> Mux13/1
  1 / rads_max/1 -> Demux13/1
  Sum18/1 -> roll_attitude/1
  Mux13/1 -> 1 / rads_max/1
  Demux16/1 -> Sum21/2
  Demux13/1 -> Sum21/1
  Sum19/1 -> roll_attitude1/1
  Mux15/1 -> 1 / rad_max/1
  [att_roll] -> Mux15/1
  roll_rate/1 -> Out1/1
  pitch_rate/1 -> Out2/1
  1 / rad_max1/1 -> Demux1/1
  Demux1/2 -> Sum19/2
  Sum1/1 -> yawl_attitude2/1
  Constant3/1 -> Sum1/2

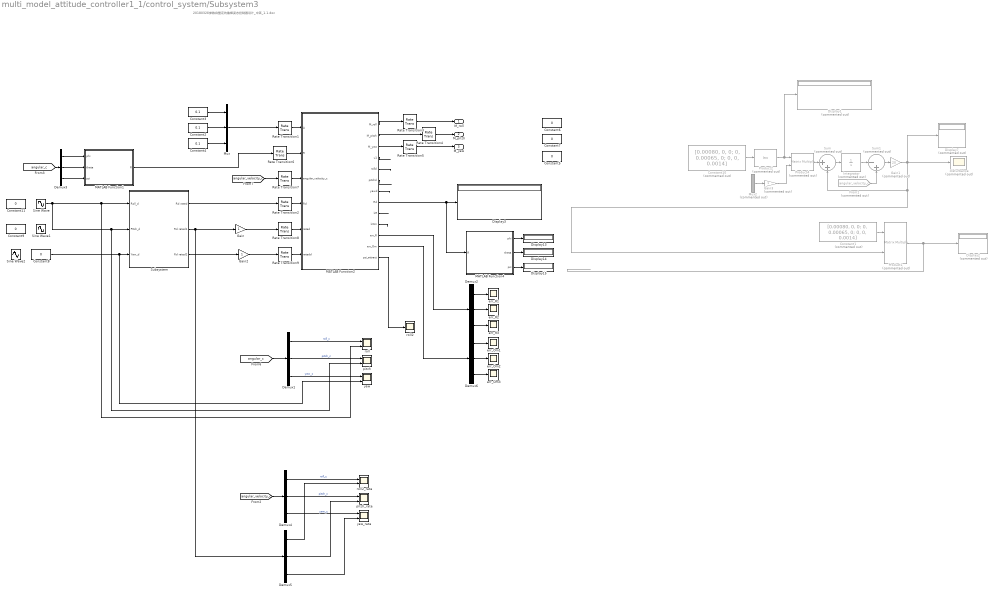
== system multi_model_attitude_controller1_1/control_system/Subsystem3 ==
  note: 20180328 参数自整定的鲁棒姿态控制器设计_中英_1.1.doc
  Constant1 : Constant  Commented=on  Value=[0.00080, 0, 0; 0, 0.00065, 0; 0, 0, 0.0014]  SampleTime=0.004
  Constant10 : Constant  Commented=on  Value=[0.00080, 0, 0; 0, 0.00065, 0; 0, 0, 0.0014]  SampleTime=0.004
  Constant{5..9,11} (6 alike) : Constant  Value=0  SampleTime=0.004
  Constant2 : Constant  Value=0.1  SampleTime=0.004
  Constant3 : Constant  Value=0.1  SampleTime=0.004
  Constant4 : Constant  Value=0.1  SampleTime=0.004
  Demux{1..6} (6 alike) : Demux  Outputs=3
  Display1 : Display  Commented=on
  Display{3,13..15} (4 alike) : Display
  Display2 : Display  Commented=on
  Display7 : Display  Commented=on
  From1 : From  Commented=on  GotoTag=angular_velocity_c  TagVisibility=global
  Gain : Gain
  Gain1 : Gain  Commented=on  Gain=20
  Gain2 : Gain
  Gain3 : Gain  Commented=on
  Integrator : Integrator  Commented=on
  MATLAB Function1 : MATLAB Function  TreatAsAtomicUnit=on
  MATLAB Function2 : MATLAB Function  TreatAsAtomicUnit=on
  MATLAB Function4 : MATLAB Function  TreatAsAtomicUnit=on
  Mux : Mux  Inputs=3
  Mux2 : Mux  Commented=on  Inputs=3
  Product1 : Product  Commented=on  Multiplication=Matrix(*)
  Product2 : Product  Commented=on  Inputs=/  Multiplication=Matrix(*)
  Product4 : Product  Commented=on  Multiplication=Matrix(*)
  Rate Transition{1..9} (9 alike) : RateTransition  OutPortSampleTime=0.004
  Sine Wave : Sin  Amplitude=pi/9  Frequency=pi  SampleTime=0.004
  Sine Wave1 : Sin  Amplitude=pi/9  Frequency=pi  Phase=pi/2  SampleTime=0.004
  Sine Wave2 : Sin  Amplitude=pi/9  Frequency=pi  SampleTime=0.004
  Subsystem : Subsystem
  Sum : Sum  Commented=on  Inputs=|++
  Sum1 : Sum  Commented=on  Inputs=|-+
  disturbance : Scope  Commented=on
  err_Om1 : Scope
  err_Om2 : Scope
  err_Om3 : Scope
  err_R1 : Scope
  err_R2 : Scope
  err_R3 : Scope
  pitch : Scope  NumInputPorts=2
  pitch_rate : Scope  NumInputPorts=2
  roll : Scope  NumInputPorts=2
  roll2 : Scope
  roll2_rate : Scope  NumInputPorts=2
  yaw : Scope  NumInputPorts=2
  yaw_rate : Scope  NumInputPorts=2
  M_roll : Outport
  M_pitch : Outport  Port=2
  M_yaw : Outport  Port=3
  wires:
  Gain3/1 -> Product4/2
  Product1/1 -> Display2/1
  Rate Transition5/1 -> M_yaw/1
  Rate Transition4/1 -> M_pitch/1
  Rate Transition3/1 -> M_roll/1
  Constant1/1 -> Product1/1
  Rate Transition2/1 -> MATLAB Function2/4("Rd ")
  Constant2/1 -> Mux/2
  From1/1 -> Sum1/2
  Gain1/1 -> Display7/1, disturbance/1, Sum/2, Product1/2
  Mux/1 -> Rate Transition1/1
  Constant10/1 -> Product2/1
  Product2/1 -> Product4/1, Display1/1
  MATLAB Function2/3(M_yaw) -> Rate Transition5/1
  Sum1/1 -> Gain1/1
  MATLAB Function2/1(M_roll) -> Rate Transition3/1
  Sum/1 -> Integrator/1
  Product4/1 -> Sum/1
  Constant3/1 -> Mux/1
  MATLAB Function2/2(M_pitch) -> Rate Transition4/1
  Subsystem/1(Rd rated) -> Rate Transition2/1
  Constant4/1 -> Mux/3
  Mux2/1 -> Gain3/1
  Integrator/1 -> Sum1/1
  Rate Transition6/1 -> MATLAB Function2/2(R)
  Demux1/3 -> yaw/1  "yaw_c"
  Rate Transition7/1 -> MATLAB Function2/3(angular_velocity_c)
  Demux1/1 -> roll/1  "roll_c"
  Rate Transition1/1 -> MATLAB Function2/1(A)
  [angular_velocity_c] -> Rate Transition7/1
  MATLAB Function1/1(R) -> Rate Transition6/1
  Demux1/2 -> pitch/1  "pitch_c"
  MATLAB Function2/5(rolld) -> ?
  MATLAB Function2/7(yawd) -> ?
  MATLAB Function2/6(pitchd) -> ?
  MATLAB Function2/4(u1) -> ?
  Demux2/1 -> err_R1/1
  MATLAB Function2/9(kR) -> ?
  MATLAB Function2/10(kOm) -> ?
  Demux2/2 -> err_R2/1
  Demux2/3 -> err_R3/1
  Constant8/1 -> yaw/2, Subsystem/3(Yaw_d)
  Sine Wave/1 -> pitch/2, Subsystem/2(PItch_d), roll/2, Subsystem/1(Roll_d)
  MATLAB Function4/1(phi) -> Display13/1
  MATLAB Function4/2(theta) -> Display14/1
  MATLAB Function4/3(psi) -> Display15/1
  MATLAB Function2/8(Rd) -> MATLAB Function4/1(R), Display3/1
  [angular_c] -> Demux1/1
  Demux3/2 -> MATLAB Function1/2(theta)
  Demux3/1 -> MATLAB Function1/1(phi)
  Demux3/3 -> MATLAB Function1/3(psi)
  Rate Transition8/1 -> MATLAB Function2/5(rated)
  Rate Transition9/1 -> MATLAB Function2/6(ratedd)
  Subsystem/2(Rd rated1) -> Demux5/1, Gain/1
  Subsystem/3(Rd rated2) -> Gain2/1
  Demux4/3 -> yaw_rate/1  "yaw_c"
  Demux4/1 -> roll2_rate/1  "roll_c"
  Demux4/2 -> pitch_rate/1  "pitch_c"
  [angular_velocity_c] -> Demux4/1
  Demux5/1 -> roll2_rate/2
  Demux5/2 -> pitch_rate/2
  Demux5/3 -> yaw_rate/2
  [angular_c] -> Demux3/1
  MATLAB Function2/13(psi_attract) -> roll2/1
  MATLAB Function2/11(err_R) -> Demux2/1
  Demux6/1 -> err_Om1/1
  Demux6/2 -> err_Om2/1
  Demux6/3 -> err_Om3/1
  MATLAB Function2/12(err_Om) -> Demux6/1
  Gain/1 -> Rate Transition8/1
  Gain2/1 -> Rate Transition9/1

== system multi_model_attitude_controller1_1/control_system1/Subsystem ==
  Add1 : Sum  Commented=on  Inputs=-+
  Add2 : Sum  Commented=on  Inputs=+-
  Constant : Constant  Commented=on  Value=[1 0 0]
  Constant1 : Constant  Commented=on  Value=[0 0 0]
  Constant11 : Constant  Value=[1; -1; 1]  SampleTime=0.004
  Constant9 : Constant  Value=[0.00080, 0, 0; 0, 0.00065, 0; 0, 0, 0.0014]  SampleTime=0.004
  Display10 : Display  Commented=on
  Display4 : Display
  Display5 : Display
  Display6 : Display
  Gain : Gain  Commented=on  Gain=1/2
  MATLAB Function3 : MATLAB Function  Commented=on  TreatAsAtomicUnit=on
  MATLAB Function4 : MATLAB Function  Commented=on  TreatAsAtomicUnit=on
  MATLAB Function5 : MATLAB Function  Commented=on  TreatAsAtomicUnit=on
  MATLAB Function7 : MATLAB Function  Commented=on  TreatAsAtomicUnit=on
  MATLAB Function8 : MATLAB Function  Commented=on  TreatAsAtomicUnit=on
  Product : Product  Inputs=/  Multiplication=Matrix(*)
  Product1 : Product  Multiplication=Matrix(*)
  Product3 : Product  Multiplication=Matrix(*)
  wires:
  ? -> Add2/1
  ? -> MATLAB Function3/1(angular)
  MATLAB Function7/1(RR) -> Add1/2
  Add1/1 -> MATLAB Function5/1(RdR_RRd)
  Constant/1 -> MATLAB Function4/1(angular)
  Gain/1 -> Display10/1  "err_R"
  MATLAB Function3/1(R) -> MATLAB Function8/1(a), MATLAB Function7/2(b)  "R"
  MATLAB Function5/1(err_R) -> Gain/1
  MATLAB Function8/1(RR) -> Add1/1
  MATLAB Function4/1(R) -> MATLAB Function8/2(b), MATLAB Function7/1(a)
  Constant1/1 -> Add2/2
  Product/1 -> Product1/1, Display5/1
  Constant11/1 -> Product3/2
  Constant9/1 -> Product3/1, Product1/2, Product/1
  Add2/1 -> ?  "err_W"
  Product3/1 -> Display6/1
  Product1/1 -> Display4/1

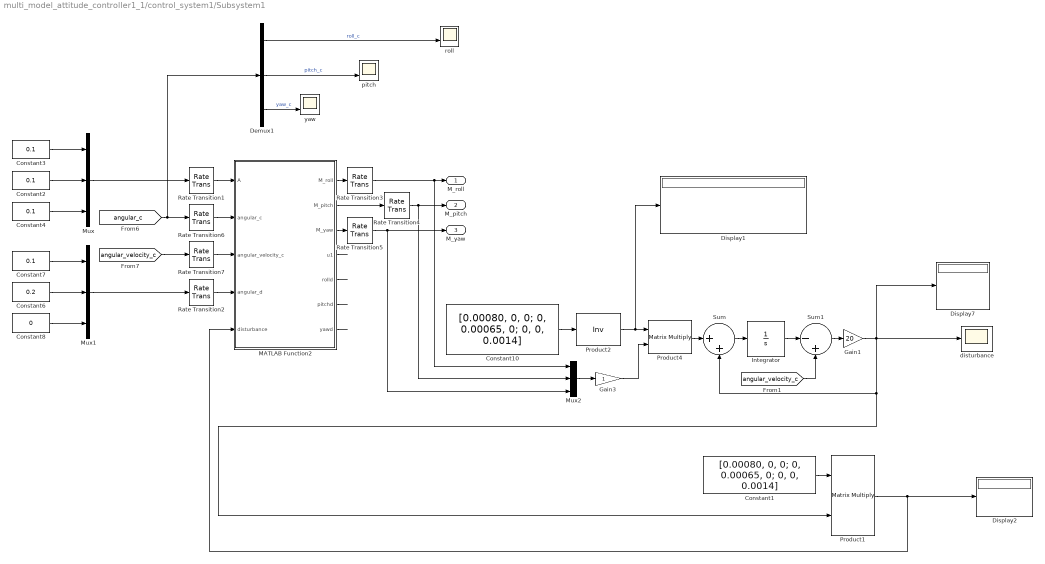
== system multi_model_attitude_controller1_1/control_system1/Subsystem1 ==
  Constant1 : Constant  Value=[0.00080, 0, 0; 0, 0.00065, 0; 0, 0, 0.0014]  SampleTime=0.004
  Constant10 : Constant  Value=[0.00080, 0, 0; 0, 0.00065, 0; 0, 0, 0.0014]  SampleTime=0.004
  Constant{2..4,7} (4 alike) : Constant  Value=0.1  SampleTime=0.004
  Constant6 : Constant  Value=0.2  SampleTime=0.004
  Constant8 : Constant  Value=0  SampleTime=0.004
  Demux1 : Demux  Outputs=3
  Display1 : Display
  Display2 : Display
  Display7 : Display
  Gain1 : Gain  Gain=20
  Gain3 : Gain
  Integrator : Integrator
  MATLAB Function2 : MATLAB Function  TreatAsAtomicUnit=on
  Mux : Mux  Inputs=3
  Mux1 : Mux  Inputs=3
  Mux2 : Mux  Inputs=3
  Product1 : Product  Multiplication=Matrix(*)
  Product2 : Product  Inputs=/  Multiplication=Matrix(*)
  Product4 : Product  Multiplication=Matrix(*)
  Rate Transition{1..7} (7 alike) : RateTransition  OutPortSampleTime=0.004
  Sum : Sum  Inputs=|++
  Sum1 : Sum  Inputs=|-+
  disturbance : Scope
  pitch : Scope  NumInputPorts=2
  roll : Scope  NumInputPorts=2
  yaw : Scope  NumInputPorts=2
  M_roll : Outport
  M_pitch : Outport  Port=2
  M_yaw : Outport  Port=3
  wires:
  MATLAB Function2/4(u1) -> ?
  MATLAB Function2/6(pitchd) -> ?
  MATLAB Function2/7(yawd) -> ?
  MATLAB Function2/5(rolld) -> ?
  ? -> pitch/1
  ? -> roll/1
  ? -> yaw/1
  Demux1/2 -> pitch/2  "pitch_c"
  [angular_c] -> Demux1/1, Rate Transition6/1
  [angular_velocity_c] -> Rate Transition7/1
  Rate Transition1/1 -> MATLAB Function2/1(A)
  Demux1/1 -> roll/2  "roll_c"
  Rate Transition7/1 -> MATLAB Function2/3(angular_velocity_c)
  Demux1/3 -> yaw/2  "yaw_c"
  Rate Transition6/1 -> MATLAB Function2/2(angular_c)
  Integrator/1 -> Sum1/1
  Mux2/1 -> Gain3/1
  Constant4/1 -> Mux/3
  Mux1/1 -> Rate Transition2/1
  MATLAB Function2/2(M_pitch) -> Rate Transition4/1
  Constant3/1 -> Mux/1
  Product4/1 -> Sum/1
  Sum/1 -> Integrator/1
  MATLAB Function2/1(M_roll) -> Rate Transition3/1
  Sum1/1 -> Gain1/1
  Constant8/1 -> Mux1/3
  MATLAB Function2/3(M_yaw) -> Rate Transition5/1
  Product2/1 -> Display1/1, Product4/1
  Constant10/1 -> Product2/1
  Mux/1 -> Rate Transition1/1
  Gain1/1 -> Product1/2, Sum/2, disturbance/1, Display7/1
  [angular_velocity_c] -> Sum1/2
  Constant6/1 -> Mux1/2
  Constant7/1 -> Mux1/1
  Constant2/1 -> Mux/2
  Rate Transition2/1 -> MATLAB Function2/4(angular_d)
  Constant1/1 -> Product1/1
  Rate Transition3/1 -> Mux2/1, M_roll/1
  Rate Transition4/1 -> Mux2/2, M_pitch/1
  Rate Transition5/1 -> Mux2/3, M_yaw/1
  Product1/1 -> MATLAB Function2/5(disturbance), Display2/1
  Gain3/1 -> Product4/2
